simulink model "RC_circuit"  (R2023a)
settings: Solver=VariableStepAuto  StartTime=0.0  StopTime=10.0  MaxStep=1e-2  RelTol=1e-3
values from neighbouring files (symbols this model uses):
  C = 1e-6    (= 1e-06)    [RC_values.m]
  R = R_vals(i)    [RC_values.m]
settings Model: Creator=EMRIX  LastModifiedBy=EMRIX

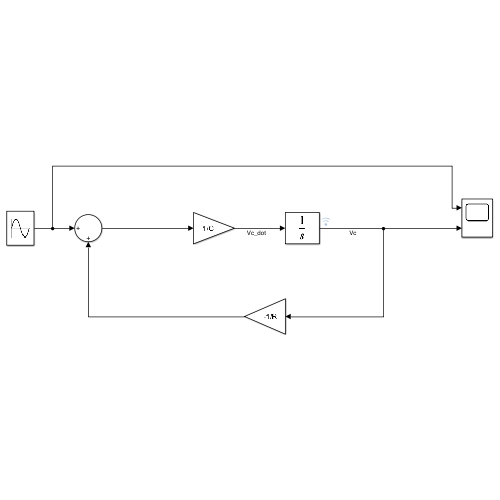
[thumbnail: Simulink's stored preview of the top-level diagram]
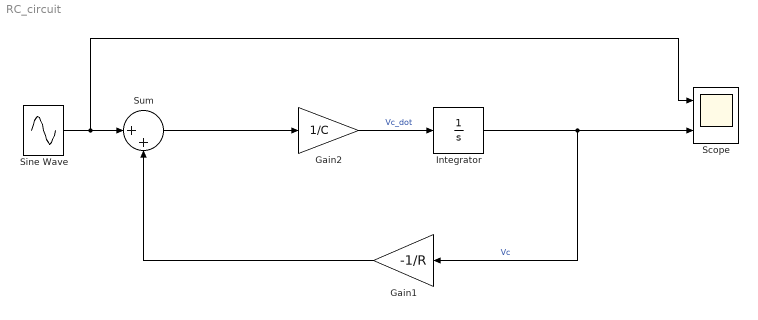
== system RC_circuit ==
  Gain1 : Gain  Gain=-1/R
  Gain2 : Gain  Gain=1/C
  Integrator : Integrator  InitialCondition=2
  Scope : Scope  NumInputPorts=2
  Sine Wave : Sin  Amplitude=5  Frequency=2*pi  SampleTime=0
  Sum : Sum  Inputs=|++
  wires:
  Gain1/1 -> Sum/2
  Sum/1 -> Gain2/1
  Integrator/1 -> Gain1/1, Scope/2  "Vc"
  Gain2/1 -> Integrator/1  "Vc_dot"
  Sine Wave/1 -> Scope/1, Sum/1
